simulink model "EjemploWebcam2017_red"  (R2016a)
settings: Solver=ode3  StartTime=0.0  StopTime=inf  FixedStep=0.01  RelTol=1e-3
libraries: LibrarySimulinkSAS x4, sldrtlib x1
settings Model: Creator=Usuario  LastModifiedBy=Usuario
settings DataIOCC: LimitDataPoints=on  SaveFormat=Array  SignalLoggingSaveFormat=ModelDataLogs
settings OptimizationCC: ExpressionDepthLimit=2147483647  SimCompilerOptimization=on
settings DebuggingCC: UnderspecifiedInitializationDetection=Classic  MergeDetectMultiDrivingBlocksExec=none  SolverPrmCheckMsg=warning  FcnCallInpInsideContextMsg=UseLocalSettings  StateNameClashWarn=warning
settings HardwareCC: ProdBitPerPointer=32  ProdLargestAtomicFloat=None  ProdIntDivRoundTo=Undefined  ProdEndianess=Unspecified  ProdWordSize=32  ProdHWDeviceType=32-bit Generic
settings ModelReferenceCC: PropagateSignalLabelsOutOfModel=off
settings GRTTargetCC: CombineOutputUpdateFcns=off  GRTInterface=on
settings ConfigComp: CovModelRefEnable=Off  CovSFcnEnable=off

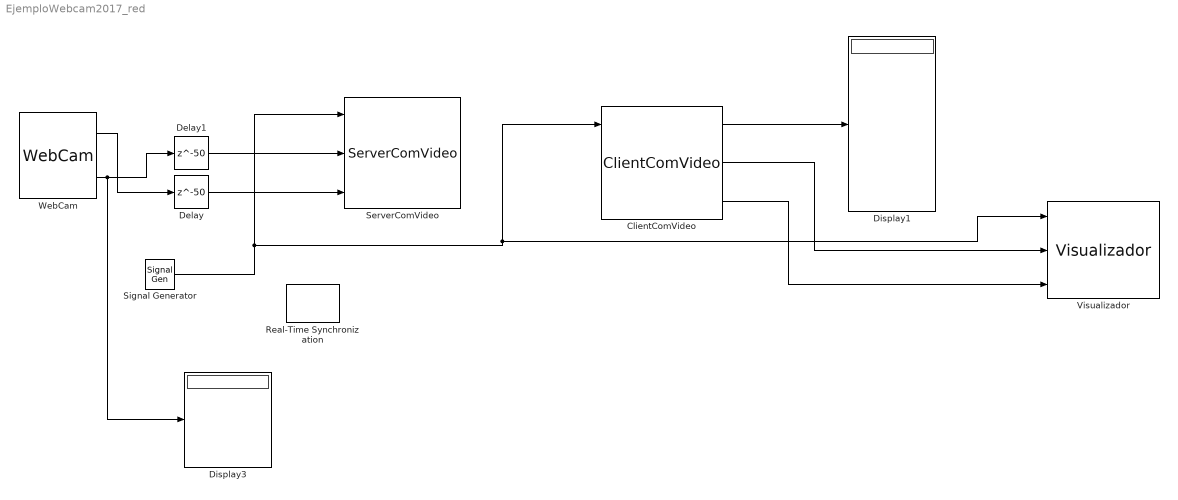
== system EjemploWebcam2017_red ==
  ClientComVideo : LibrarySimulinkSAS/ClientComVideo
  Delay : Delay  DelayLength=50
  Delay1 : Delay  DelayLength=50
  Display1 : Display
  Display3 : Display
  Real-Time Synchronization : sldrtlib/Real-Time Synchronization  SampleTime=0.1  MaxMissedTicks=inf  ShowMissedTicks=off  YieldWhenWaiting=off
  ServerComVideo : LibrarySimulinkSAS/ServerComVideo
  Signal Generator : SignalGenerator  WaveForm=square  Frequency=10
  Visualizador : LibrarySimulinkSAS/Visualizador
  WebCam : LibrarySimulinkSAS/WebCam
  wires:
  Signal Generator/1 -> Visualizador/1, ClientComVideo/1, ServerComVideo/1
  ClientComVideo/1 -> Display1/1
  ClientComVideo/3 -> Visualizador/3
  ClientComVideo/2 -> Visualizador/2
  WebCam/1 -> Delay/1
  Delay/1 -> ServerComVideo/3
  WebCam/2 -> Display3/1, Delay1/1
  Delay1/1 -> ServerComVideo/2
